simulink model "NEWEST"  (R2024b)
settings: Solver=ode1  StartTime=0.0  StopTime=inf  FixedStep=0.002  RelTol=1e-3  EnableMultiTasking=on
libraries: me375_robot x4
settings Model: SimulationMode=external  ExtModeTrigDuration=2  Creator=gc90s  LastModifiedBy=gc90s
settings SolverCC: AutoInsertRateTranBlk=on
settings OptimizationCC: EnhancedBackFolding=on  PassReuseOutputArgsAs=Individual arguments  ZeroExternalMemoryAtStartup=off  ZeroInternalMemoryAtStartup=off  MaxStackSize=64  OptimizeBlockOrder=speed  DifferentSizesBufferReuse=on  EfficientTunableParamExpr=on
settings DebuggingCC: ParameterPrecisionLossMsg=none  ParameterTunabilityLossMsg=error
settings HardwareCC: ProdBitPerInt=16  ProdBitPerPointer=16  ProdBitPerSizeT=16  ProdBitPerPtrDiffT=16  ProdLargestAtomicFloat=None  ProdWordSize=8  ProdHWDeviceType=Atmel->AVR  UseEmbeddedCoderFeatures=off  UseSimulinkCoderFeatures=off
settings SFSimCC: MATLABDynamicMemAlloc=off
settings RTWCC: Description=Embedded Coder  SystemTargetFile=ert.tlc  HardwareBoard=Arduino Mega 2560  TemplateMakefile=ert_default_tmf  Toolchain=Arduino AVR  BuildConfiguration=Faster Runs
settings CodeAppCC: ForceParamTrailComments=on  IgnoreCustomStorageClasses=off  OperatorAnnotations=on  SimulinkDataObjDesc=on  SFDataObjDesc=on  MangleLength=10  InsertBlockDesc=on
settings ERTTargetCC: SupportContinuousTime=on  SupportNonInlinedSFcns=on  SupportVariableSizeSignals=on  ExtModeTransport=3  ExtModeStaticAlloc=on  ExtModeAutomaticAllocSize=off  ExtModeStaticAllocSize=2048  ExtModeMexFile=ext_xcp  ExtModeIntrfLevel=Level2 - Open  InlinedParameterPlacement=Hierarchical

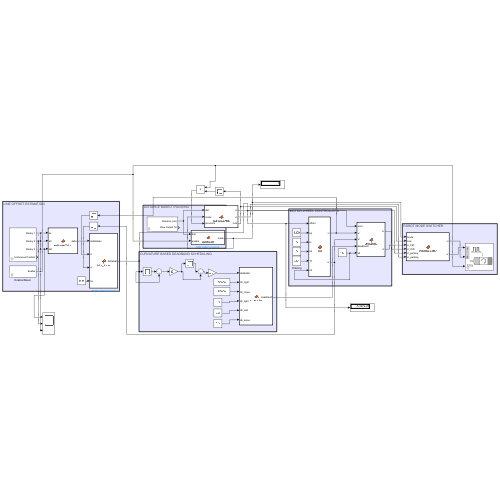
[thumbnail: Simulink's stored preview of the top-level diagram]
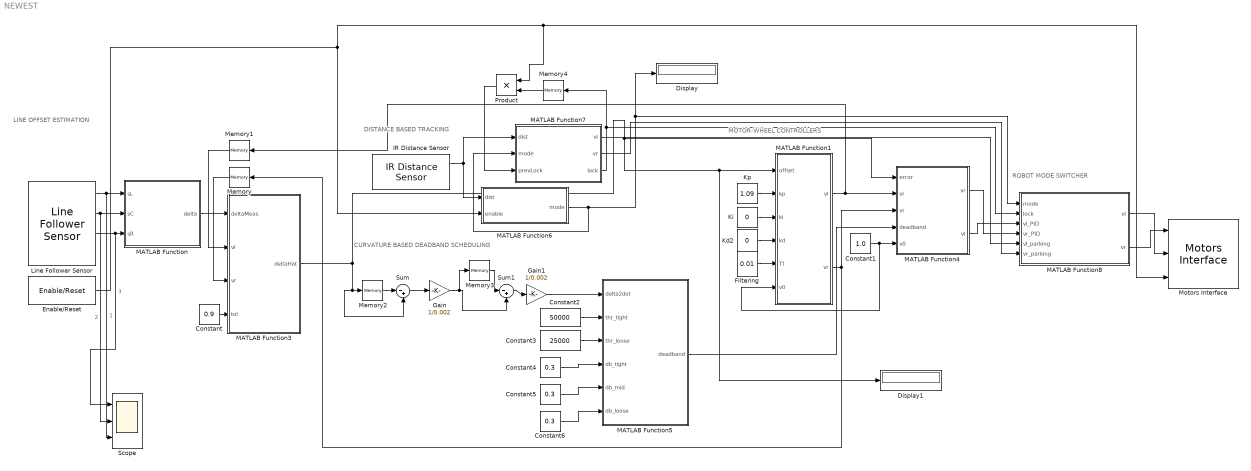
== system NEWEST ==
  note: ROBOT MODE SWITCHER
  note: MOTOR-WHEEL CONTROLLERS
  note: DISTANCE BASED TRACKING
  note: CURVATURE BASED DEADBAND SCHEDULING
  note: LINE OFFSET ESTIMATION
  Constant : Constant  Value=0.9
  Constant1 : Constant  Value=1.0
  Constant2 : Constant  Value=50000
  Constant3 : Constant  Value=25000
  Constant4 : Constant  Value=0.3
  Constant5 : Constant  Value=0.3
  Constant6 : Constant  Value=0.3
  Display : Display
  Display1 : Display
  Enable/Reset : me375_robot/Enable//Reset  PinEnable=20  enable_override=off
      settings: SourceProductName=ME 375 Robot Project
  Filtering : Constant  Value=0.01
  Gain : Gain  Gain=1/0.002
  Gain1 : Gain  Gain=1/0.002
  IR Distance Sensor : me375_robot/IR Distance Sensor  pinNumber=0  CalibValsEnabled=off  Gain4=-4.3019  Gain5=239.1904  Gain6=-0.6848  Gain7=48.1191
      settings: SourceProductName=ME 375 Robot Project
  Kd2 : Constant  Value=0
  Ki : Constant  Value=0
  Kp : Constant  Value=1.09
  Line Follower Sensor : me375_robot/Line Follower Sensor  Value=400  cont_thresh=256
      settings: SourceProductName=ME 375 Robot Project
  MATLAB Function : MATLAB Function  TreatAsAtomicUnit=on
  MATLAB Function1 : MATLAB Function  TreatAsAtomicUnit=on
  MATLAB Function3 : MATLAB Function  TreatAsAtomicUnit=on
  MATLAB Function4 : MATLAB Function  TreatAsAtomicUnit=on
  MATLAB Function5 : MATLAB Function  TreatAsAtomicUnit=on
  MATLAB Function6 : MATLAB Function  TreatAsAtomicUnit=on
  MATLAB Function7 : MATLAB Function  TreatAsAtomicUnit=on
  MATLAB Function8 : MATLAB Function  TreatAsAtomicUnit=on
  Memory{,1..4} (5 alike) : Memory
  Motors Interface : me375_robot/Motors Interface  Value=1  pinNumber0=6  pinNumber2=7  pinNumber1=8  pinNumber3=9  desiredFrequency=31372.55
      settings: SourceProductName=ME 375 Robot Project
  Product : Product
  Scope : Scope  NumInputPorts=3
  Sum : Sum  Inputs=|-+
  Sum1 : Sum  Inputs=|-+
  wires:
  Line Follower Sensor/2 -> MATLAB Function/2(sC), Scope/2  "2"
  Line Follower Sensor/1 -> Scope/3, MATLAB Function/1(sL)  "1"
  Line Follower Sensor/3 -> Scope/1, MATLAB Function/3(sR)  "3"
  Enable/Reset/1 -> MATLAB Function6/2(enable), Product/1, Motors Interface/3
  Filtering/1 -> MATLAB Function1/5(Tf)
  MATLAB Function/1(delta) -> MATLAB Function3/1(deltaMeas)
  MATLAB Function1/2(vr) -> MATLAB Function4/3("vr "), Memory/1
  MATLAB Function1/1(vl) -> MATLAB Function4/2("vl "), Memory1/1
  Constant1/1 -> MATLAB Function4/5(v0), MATLAB Function1/6(v0)
  MATLAB Function5/1(deadband) -> MATLAB Function4/4(deadband)
  Kd2/1 -> MATLAB Function1/4(kd)
  Kp/1 -> MATLAB Function1/2(kp)
  MATLAB Function3/1(deltaHat) -> MATLAB Function4/1(error), Display1/1, MATLAB Function1/1(offset), Sum/2, Memory2/1
  Constant/1 -> MATLAB Function3/4(tol)
  Ki/1 -> MATLAB Function1/3(ki)
  Memory1/1 -> MATLAB Function3/2(vl)
  Memory/1 -> MATLAB Function3/3(vr)
  Memory2/1 -> Sum/1
  Sum/1 -> Gain/1
  Gain/1 -> Sum1/2, Memory3/1
  Memory3/1 -> Sum1/1
  Sum1/1 -> Gain1/1
  Gain1/1 -> MATLAB Function5/1(delta2dot)
  Constant2/1 -> MATLAB Function5/2(thr_tight)
  Constant3/1 -> MATLAB Function5/3(thr_loose)
  Constant4/1 -> MATLAB Function5/4(db_tight)
  Constant5/1 -> MATLAB Function5/5(db_mid)
  Constant6/1 -> MATLAB Function5/6(db_loose)
  IR Distance Sensor/1 -> MATLAB Function7/1(dist), MATLAB Function6/1(dist)
  MATLAB Function6/1(mode) -> MATLAB Function7/2(mode), Display/1, MATLAB Function8/1(mode)
  MATLAB Function7/1(vl) -> MATLAB Function8/5(vl_parking)
  MATLAB Function7/2(vr) -> MATLAB Function8/6(vr_parking)
  MATLAB Function8/2(vr) -> Motors Interface/1
  MATLAB Function8/1(vl) -> Motors Interface/2
  MATLAB Function4/2(vl) -> MATLAB Function8/3(vl_PID)
  MATLAB Function4/1(vr) -> MATLAB Function8/4(vr_PID)
  MATLAB Function7/3(lock) -> Memory4/1, MATLAB Function8/2(lock)
  Memory4/1 -> Product/2
  Product/1 -> MATLAB Function7/3(prevLock)

== matlab function NEWEST/MATLAB Function1 ==
  settings: updateMethod=DISCRETE
  data: vl output; vr output; offset input; kp input; ki input; kd input; Tf input; v0 input
function [vl, vr] = pid(offset, kp, ki, kd, Tf, v0)
% … [header unchanged] …

vMax = 1.0;              % actuator limits
Ts   = 0.002;            % sample time
persistent I errPrev dFilt
if isempty(I), I = 0; errPrev = 0; dFilt = 0; end

% ----- PID -------------------------------------------------------------
err = offset;
I    = I + ki*err*Ts;                         % integral
dRaw = (err - errPrev)/Ts;                    % derivative (raw)

alpha = Tf/(Tf+Ts);                           % LPF on D
dFilt = alpha*dFilt + (1-alpha)*dRaw;
D     = kd*dFilt;

u  = kp*err + I + D;                          % steering before sat
u  = min(max(u,-vMax), vMax);                 % saturate steering

% anti-wind-up
if abs(u)==vMax, I = I - ki*err*Ts; end

% ----- raw wheel speeds ------------------------------------------------
vl_raw =  v0 - u;
vr_raw =  v0 + u;

% ----- NEW: scale so that max(|vl|,|vr|) == vMax -----------------------
m      = max(abs(vl_raw), abs(vr_raw));
if m < vMax && m > 0                        % only scale up
    s       = vMax/m;                       % scale factor ≥ 1
    vl_raw  = vl_raw * s;
    vr_raw  = vr_raw * s;
end

% ----- final saturation (safety) ---------------------------------------
vl = min(max(vl_raw,-vMax), vMax);
vr = min(max(vr_raw,-vMax), vMax);

errPrev = err;
end

== matlab function NEWEST/MATLAB Function ==
  settings: updateMethod=DISCRETE
  data: sL input; delta output; sC input; sR input
function delta = estimateDelta(sL, sC, sR)
%ESTIMATEDELTA  Convert 3 digital reflectance readings to lateral offset δ
%   sL,sC,sR : left, centre, right (1 = black, 0 = white)
%   delta    : signed offset [inch] (+ right, – left)
%
% Geometry (exact from drawing)
w = 23.5/64;          % stripe width               [in]
g = 5/64;             % gap between stripes        [in]
d = 3/8;              % sensor spacing             [in]
% Pre-computed mid-points of admissible intervals (see table above)
persistent LUT lastDelta
if isempty(LUT)
    LUT = nan(8,1);               % index = sL*4 + sC*2 + sR
    LUT(bin2dec('001')+1) = -0.598;            % only R black
    LUT(bin2dec('011')+1) = -0.188;            % C & R black
    LUT(bin2dec('010')+1) =  0.371;            % only C black
    LUT(bin2dec('101')+1) =  0.000;            % L & R black (centre)
    LUT(bin2dec('110')+1) =  0.188;            % L & C black
    LUT(bin2dec('100')+1) =  0.598;            % only L black
    % LUT(000) and LUT(111) stay NaN → “lost” / impossible
    lastDelta = 0;
end

idx   = 4*sL + 2*sC + sR;         % binary → 0…7
delta = LUT(idx+1);

% Handle ambiguous / lost patterns
switch idx
    case bin2dec('010')            % only centre black: sign unknown
        if lastDelta < 0
            delta = -abs(delta);
        else
            delta =  abs(delta);
        end
    otherwise
        if isnan(delta)            % 000, 111, or any undefined state
            delta = lastDelta;     % hold the most recent finite value
        end
end

lastDelta = delta;                 % remember for next call
end

== matlab function NEWEST/MATLAB Function3 ==
  data: deltaMeas input; deltaHat output; vl input; vr input; tol input
function deltaHat = delta_fusion(deltaMeas, vl, vr, tol)
% deltaMeas : output of estimateDelta (NaN when 000 pattern)
% vl,vr     : wheel speeds  (-1…1)   [command units]
% deltaHat  : fused, continuous lateral error [in]
%
% Tunables
B     = 6.5;       % wheel-base          [in]  (measure yours!)
Ts    = 0.002;     % sample time         [s]
Ksens = tol;      % 0 = ignore sensors, 1 = full trust

persistent x
if isempty(x), x = 0; end            % initial δ̂

% dead-reckon lateral motion (small-angle approx)
xPred = x + ((vr - vl)/B)*Ts;

% sensor correction if valid
if ~isnan(deltaMeas)
    x = xPred + Ksens*(deltaMeas - xPred);
else
    x = xPred;
end

deltaHat = x;
end

== matlab function NEWEST/MATLAB Function4 ==
  data: error input; vr output; vl input; vr input; deadband input; v0 input; vl output
function [vr, vl] = deadband(error, vl, vr, deadband, v0)
    if abs(error) <= deadband
        vl = v0;
        vr = v0;
    end

== matlab function NEWEST/MATLAB Function5 ==
  data: delta2dot input; deadband output; thr_tight input; thr_loose input; db_tight input; db_mid input; db_loose input
function deadband = scheduler(delta2dot,...
                                        thr_tight, thr_loose,...
                                        db_tight, db_mid, db_loose)
%DEADBAND_SCHEDULER   Pick dead-band value from curvature “jerk”.
%
% States
%   0  = STRAIGHT       (|δ̈| < thr_loose   for ≥ τ_loose)
%   1  = GENTLE BEND    (in between)
%   2  = TIGHT TURN     (|δ̈| > thr_tight   for ≥ τ_tight)
%
% INPUTS
%   delta2dot   – second derivative of δ  [in·s⁻²]
%   Ts          – sample time             [s]   (e.g. 0.002)
%   thr_tight   – |δ̈| threshold to enter state 2
%   thr_loose   – |δ̈| threshold to leave  state 2  (hysteresis)
%   db_tight    – dead-band in state 2    [in]
%   db_mid      – dead-band in state 1    [in]
%   db_loose    – dead-band in state 0    [in]
%
% OUTPUT
%   deadband    – selected dead-band      [in]

Ts = 0.002;
deadband = db_tight;

% ─── persistent state ────────────────────────────────────────────────
persistent state tHigh tLow filt
if isempty(state)
    [state,tHigh,tLow,filt] = deal(0,0,0,0);
end

% ─── 1.  Low-pass filter to tame noise (1st-order, fc≈10 Hz) ─────────
alpha = exp(-2*pi*5*Ts);           % pole @ 10 Hz
filt  = alpha*filt + (1-alpha)*abs(delta2dot);

% ─── 2.  State machine with dwell times (hysteresis) ─────────────────
tau_tight = 0.04;   % 20 ms above thr_tight to confirm tight turn
tau_loose = 0.02;   % 40 ms below thr_loose to re-enter straight

switch state
    case 0   % ── STRAIGHT ───────────────────────────────────────────
        if filt > thr_tight
            tHigh = 0;  state = 1;  % first go to intermediate
        end

    case 1   % ── GENTLE BEND ----------------------------------------
        if filt > thr_tight
            tHigh = tHigh + Ts;
            if tHigh >= tau_tight
                state = 2;          % confirmed tight turn
            end
        elseif filt < thr_loose
            tLow = tLow + Ts;
            if tLow >= tau_loose
                state = 0;          % back to straight
            end
        else
            tHigh = 0;  tLow = 0;   % reset dwell counters
        end

    case 2   % ── TIGHT TURN -----------------------------------------
        if filt < thr_loose
            tLow = tLow + Ts;
            if tLow >= tau_loose
                state = 1;          % relax to gentle bend first
            end
        else
            tLow = 0;
        end
end

% ─── 3.  Output the corresponding dead-band ─────────────────────────
switch state
    case 0, deadband = db_loose;   % straight
    case 1, deadband = db_mid;     % gentle bend
    case 2, deadband = db_tight;   % tight turn
end
end

== matlab function NEWEST/MATLAB Function6 ==
  settings: updateMethod=DISCRETE
  data: dist input; mode output; enable input
function mode = lidarMode(dist, enable)

    if dist <= 8 && enable == 1
        mode = 1;
    else
        mode = 0;
    end

end

== matlab function NEWEST/MATLAB Function7 ==
  data: dist input; vl output; vr output; mode input; lock output; prevLock input
function [vl, vr, lock] = parkingControl(dist, mode, prevLock)
    % dist in meters
    if prevLock == 1 || mode == 1
        lock = 1;
        v_reverse = -0.3;   % reverse speed (adjust as needed)
        stopDist  = 20.3;   % stop at 20 cm
        margin    = 0.1;   % small tolerance
        
        if dist < stopDist - margin
            speed = v_reverse;
        else
            speed = 0;
        end
        
        vl = speed;
        vr = speed;
    else
        lock = 0;
        vl = 0;
        vr = 0;
    end
    
end

== matlab function NEWEST/MATLAB Function8 ==
  data: mode input; lock input; vl output; vl_PID input; vr_PID input; vl_parking input; vr_parking input; vr output
function [vl, vr] = modeSelector(mode, lock, vl_PID, vr_PID, vl_parking, vr_parking)
    if lock == 1 || mode == 1
        vl = vl_parking;
        vr = vr_parking;
    else
        vl = vl_PID;
        vr = vr_PID;
    end
end
